simulink model "ENV_scheduled"  (R2024b)
settings: Solver=FixedStepDiscrete  StartTime=0.0  StopTime=10.0  FixedStep=0.001  RelTol=1e-3
libraries: stm32blockslib x54, canmsglib x29, simulink x7, stm32f4xxblockslib x1
(part 4 of 5)

== system ENV_scheduled/CAN Tx7 ==
  MCPInitialized : Inport  SampleTime=.001
  BBMSP0A0E : Inport  Port=2
  BBMSP0A10 : Inport  Port=3
  MTorqueVectoringFL : Inport  Port=4
  MTorqueVectoringFR : Inport  Port=5
  MTorqueVectoringRL : Inport  Port=6
  MTorqueVectoringRR : Inport  Port=7
  NTractionControlMultiplierFL : Inport  Port=8
  NTractionControlMultiplierFR : Inport  Port=9
  Bus Selector : BusSelector  OutputSignals=ID,Length,Data
  CAN Pack : canmsglib/CAN Pack  CANdbFile=C:\Users\William\Downloads\VCUSTM32\BaselineControls\CAN\CAN3_baseline.dbc  MsgList=Etas_Signals_08  MsgName=Etas_Signals_08  MsgIDType=Standard (11-bit identifier)  MsgIdentifier=2036  CANIDInput=off  MsgLength=8  Remote=off  ApplyMinMax=off  BusOutput=on  SignalInfo={'BBMSP0A0E','62','1','LE','unsigned','Standard','0','1','0','0','1';'BBMSP0A10','63','1','LE','unsigned','Standard','0','1','0','0','1';'MTorqueVectoringFL','12','12','LE','signed','Standard','0','0.1','50','-154.8','254.7';'MTorqueVectoringFR','24','12','LE','signed','Standard','0','0.1','50','-154.8','254.7';'MTorqueVectoringRL','36','12','LE','signed','Standard','0','0.1','50','-154.8','254.7';'MTorqueVectoringRR','0','12','LE','signed','Standard','0','0.1','50','-154.8','254.7';'NTractionControlMultiplierFL','55','7','LE','unsigned','Standard','0','0.01','0','0','1.27';'NTractionControlMultiplierFR','48','7','LE','unsigned','Standard','0','0.01','0','0','1.27'}
      settings: LibrarySourceBlock=stmutilitieslib/CAN Pack  DataFormat=CANdb specified signals
  MATLAB Function : MATLAB Function  TreatAsAtomicUnit=on
  Offset : Constant  Value=3  OutDataTypeStr=uint16  SampleTime=.001
  Period : Constant  Value=20  OutDataTypeStr=uint16  SampleTime=.001
  RTS : Constant  Value=0x82  OutDataTypeStr=uint8  SampleTime=.001
  SPI Controller Transfer : stm32blockslib/SPI Controller Transfer  Priority=1  SPIModuleSelect=SPI1  ClockPolarity=Low  ClockPhase=1 Edge  SPIModule=uint32(0)  Mode=Master  BusSpeed=uint32(1000000)  FirstBitToTransfer=Most significant bit (MSB)  ClockMode=0  BlockFunction=Transfer  EnableRegisterAddress=off  RegisterAddress=0  OutputDataType=uint8  OutputDataLength=1  OutputStatus=off  BlockingMode=off  Timeout=0.01  DataBits=8  UseCustomSSPin=Explicit GPIO calls  ActiveLowSSPin=Active low  Port_Select=GPIOA  Pin=4
      settings: LibrarySourceBlock=stm32h7xxblockslib/SPI Controller Transfer
  SPI Controller Transfer1 : stm32blockslib/SPI Controller Transfer  Priority=2  SPIModuleSelect=SPI1  ClockPolarity=Low  ClockPhase=1 Edge  SPIModule=uint32(0)  Mode=Master  BusSpeed=uint32(1000000)  FirstBitToTransfer=Most significant bit (MSB)  ClockMode=0  BlockFunction=Transfer  EnableRegisterAddress=off  RegisterAddress=0  OutputDataType=uint8  OutputDataLength=1  OutputStatus=off  BlockingMode=off  Timeout=0.01  DataBits=8  UseCustomSSPin=Explicit GPIO calls  ActiveLowSSPin=Active low  Port_Select=GPIOA  Pin=4
      settings: LibrarySourceBlock=stm32h7xxblockslib/SPI Controller Transfer
  TX Buffer 0 : Constant  Value=0x41  OutDataTypeStr=uint8  SampleTime=.001
  Terminator : Terminator
  Terminator1 : Terminator
  Vector Concatenate : Concatenate  NumInputs=3
  wires:
  BBMSP0A10/1 -> CAN Pack/2
  BBMSP0A0E/1 -> CAN Pack/1
  MTorqueVectoringFL/1 -> CAN Pack/3
  MTorqueVectoringFR/1 -> CAN Pack/4
  MTorqueVectoringRL/1 -> CAN Pack/5
  MTorqueVectoringRR/1 -> CAN Pack/6
  NTractionControlMultiplierFL/1 -> CAN Pack/7
  NTractionControlMultiplierFR/1 -> CAN Pack/8
  RTS/1 -> MATLAB Function/4(RTS)
  MATLAB Function/1(WriteInstruction) -> Vector Concatenate/1
  TX Buffer 0/1 -> Vector Concatenate/2
  SPI Controller Transfer1/1 -> Terminator1/1
  MATLAB Function/2(CANVector) -> Vector Concatenate/3
  Offset/1 -> MATLAB Function/6(offset)
  Bus Selector/2 -> MATLAB Function/2(Length)  "<Length>"
  Bus Selector/3 -> MATLAB Function/3(Data)  "<Data>"
  Vector Concatenate/1 -> SPI Controller Transfer/1
  MCPInitialized/1 -> MATLAB Function/7(MCPInitialized)
  Period/1 -> MATLAB Function/5(period)
  Bus Selector/1 -> MATLAB Function/1(ID)  "<ID>"
  CAN Pack/1 -> Bus Selector/1
  SPI Controller Transfer/1 -> Terminator/1
  MATLAB Function/3(RTSByte) -> SPI Controller Transfer1/1

== system ENV_scheduled/CAN Tx8 ==
  MCPInitialized : Inport  SampleTime=.001
  MDischargeLimited : Inport  Port=2
  MDriverRegenRequested : Inport  Port=3
  MRegenLimited : Inport  Port=4
  MSpinningModelFL : Inport  Port=5
  MSpinningModelFR : Inport  Port=6
  NCarState : Inport  Port=7
  rSlipRatioOptimal : Inport  Port=8
  Bus Selector : BusSelector  OutputSignals=ID,Length,Data
  CAN Pack : canmsglib/CAN Pack  CANdbFile=C:\Users\William\Downloads\VCUSTM32\BaselineControls\CAN\CAN3_baseline.dbc  MsgList=Etas_Signals_09  MsgName=Etas_Signals_09  MsgIDType=Standard (11-bit identifier)  MsgIdentifier=2037  CANIDInput=off  MsgLength=8  Remote=off  ApplyMinMax=off  BusOutput=on  SignalInfo={'MDischargeLimited','0','13','LE','unsigned','Standard','0','0.1','0','0','819.1';'MDriverRegenRequested','13','11','LE','unsigned','Standard','0','-0.1','0','-204.7','0';'MRegenLimited','30','11','LE','unsigned','Standard','0','-0.1','0','-204.7','0';'MSpinningModelFL','41','8','LE','unsigned','Standard','0','0.1','0','-Inf','Inf';'MSpinningModelFR','49','8','LE','unsigned','Standard','0','0.1','0','-Inf','Inf';'NCarState','57','7','LE','unsigned','Standard','0','1','0','0','127';'rSlipRatioOptimal','24','6','LE','unsigned','Standard','0','0.01','0','0','0.63'}
      settings: LibrarySourceBlock=stmutilitieslib/CAN Pack  DataFormat=CANdb specified signals
  MATLAB Function : MATLAB Function  TreatAsAtomicUnit=on
  Offset : Constant  Value=3  OutDataTypeStr=uint16  SampleTime=.001
  Period : Constant  Value=20  OutDataTypeStr=uint16  SampleTime=.001
  RTS : Constant  Value=0x84  OutDataTypeStr=uint8  SampleTime=.001
  SPI Controller Transfer : stm32blockslib/SPI Controller Transfer  Priority=1  SPIModuleSelect=SPI1  ClockPolarity=Low  ClockPhase=1 Edge  SPIModule=uint32(0)  Mode=Master  BusSpeed=uint32(1000000)  FirstBitToTransfer=Most significant bit (MSB)  ClockMode=0  BlockFunction=Transfer  EnableRegisterAddress=off  RegisterAddress=0  OutputDataType=uint8  OutputDataLength=1  OutputStatus=off  BlockingMode=off  Timeout=0.01  DataBits=8  UseCustomSSPin=Explicit GPIO calls  ActiveLowSSPin=Active low  Port_Select=GPIOA  Pin=4
      settings: LibrarySourceBlock=stm32h7xxblockslib/SPI Controller Transfer
  SPI Controller Transfer1 : stm32blockslib/SPI Controller Transfer  Priority=2  SPIModuleSelect=SPI1  ClockPolarity=Low  ClockPhase=1 Edge  SPIModule=uint32(0)  Mode=Master  BusSpeed=uint32(1000000)  FirstBitToTransfer=Most significant bit (MSB)  ClockMode=0  BlockFunction=Transfer  EnableRegisterAddress=off  RegisterAddress=0  OutputDataType=uint8  OutputDataLength=1  OutputStatus=off  BlockingMode=off  Timeout=0.01  DataBits=8  UseCustomSSPin=Explicit GPIO calls  ActiveLowSSPin=Active low  Port_Select=GPIOA  Pin=4
      settings: LibrarySourceBlock=stm32h7xxblockslib/SPI Controller Transfer
  TX Buffer 0 : Constant  Value=0x51  OutDataTypeStr=uint8  SampleTime=.001
  Terminator : Terminator
  Terminator1 : Terminator
  Vector Concatenate : Concatenate  NumInputs=3
  wires:
  MDriverRegenRequested/1 -> CAN Pack/2
  MDischargeLimited/1 -> CAN Pack/1
  MRegenLimited/1 -> CAN Pack/3
  MSpinningModelFL/1 -> CAN Pack/4
  MSpinningModelFR/1 -> CAN Pack/5
  NCarState/1 -> CAN Pack/6
  rSlipRatioOptimal/1 -> CAN Pack/7
  CAN Pack/1 -> Bus Selector/1
  SPI Controller Transfer/1 -> Terminator/1
  Bus Selector/1 -> MATLAB Function/1(ID)  "<ID>"
  Period/1 -> MATLAB Function/5(period)
  Bus Selector/3 -> MATLAB Function/3(Data)  "<Data>"
  Vector Concatenate/1 -> SPI Controller Transfer/1
  Bus Selector/2 -> MATLAB Function/2(Length)  "<Length>"
  Offset/1 -> MATLAB Function/6(offset)
  SPI Controller Transfer1/1 -> Terminator1/1
  MATLAB Function/2(CANVector) -> Vector Concatenate/3
  TX Buffer 0/1 -> Vector Concatenate/2
  MATLAB Function/3(RTSByte) -> SPI Controller Transfer1/1
  RTS/1 -> MATLAB Function/4(RTS)
  MCPInitialized/1 -> MATLAB Function/7(MCPInitialized)
  MATLAB Function/1(WriteInstruction) -> Vector Concatenate/1

== system ENV_scheduled/CAN Tx9 ==
  MCPInitialized : Inport  SampleTime=.001
  MSpinningModelRL : Inport  Port=2
  MSpinningModelRR : Inport  Port=3
  MTorqueDistributionFL : Inport  Port=4
  MTorqueDistributionFR : Inport  Port=5
  MTorqueDistributionRL : Inport  Port=6
  MTorqueDistributionRR : Inport  Port=7
  Bus Selector : BusSelector  OutputSignals=ID,Length,Data
  CAN Pack : canmsglib/CAN Pack  CANdbFile=C:\Users\William\Downloads\VCUSTM32\BaselineControls\CAN\CAN3_baseline.dbc  MsgList=Etas_Signals_10  MsgName=Etas_Signals_10  MsgIDType=Standard (11-bit identifier)  MsgIdentifier=2038  CANIDInput=off  MsgLength=8  Remote=off  ApplyMinMax=off  BusOutput=on  SignalInfo={'MSpinningModelRL','8','8','LE','unsigned','Standard','0','0.1','0','-Inf','Inf';'MSpinningModelRR','0','8','LE','unsigned','Standard','0','0.1','0','0','25.5';'MTorqueDistributionFL','40','12','LE','signed','Standard','0','0.1','50','-154.8','254.7';'MTorqueDistributionFR','16','12','LE','signed','Standard','0','0.1','50','-154.8','254.7';'MTorqueDistributionRL','52','12','LE','signed','Standard','0','0.1','50','-154.8','254.7';'MTorqueDistributionRR','28','12','LE','signed','Standard','0','0.1','50','-154.8','254.7'}
      settings: LibrarySourceBlock=stmutilitieslib/CAN Pack  DataFormat=CANdb specified signals
  MATLAB Function : MATLAB Function  TreatAsAtomicUnit=on
  Offset : Constant  Value=4  OutDataTypeStr=uint16  SampleTime=.001
  Period : Constant  Value=20  OutDataTypeStr=uint16  SampleTime=.001
  RTS : Constant  Value=0x81  OutDataTypeStr=uint8  SampleTime=.001
  SPI Controller Transfer : stm32blockslib/SPI Controller Transfer  Priority=1  SPIModuleSelect=SPI1  ClockPolarity=Low  ClockPhase=1 Edge  SPIModule=uint32(0)  Mode=Master  BusSpeed=uint32(1000000)  FirstBitToTransfer=Most significant bit (MSB)  ClockMode=0  BlockFunction=Transfer  EnableRegisterAddress=off  RegisterAddress=0  OutputDataType=uint8  OutputDataLength=1  OutputStatus=off  BlockingMode=off  Timeout=0.01  DataBits=8  UseCustomSSPin=Explicit GPIO calls  ActiveLowSSPin=Active low  Port_Select=GPIOA  Pin=4
      settings: LibrarySourceBlock=stm32h7xxblockslib/SPI Controller Transfer
  SPI Controller Transfer1 : stm32blockslib/SPI Controller Transfer  Priority=2  SPIModuleSelect=SPI1  ClockPolarity=Low  ClockPhase=1 Edge  SPIModule=uint32(0)  Mode=Master  BusSpeed=uint32(1000000)  FirstBitToTransfer=Most significant bit (MSB)  ClockMode=0  BlockFunction=Transfer  EnableRegisterAddress=off  RegisterAddress=0  OutputDataType=uint8  OutputDataLength=1  OutputStatus=off  BlockingMode=off  Timeout=0.01  DataBits=8  UseCustomSSPin=Explicit GPIO calls  ActiveLowSSPin=Active low  Port_Select=GPIOA  Pin=4
      settings: LibrarySourceBlock=stm32h7xxblockslib/SPI Controller Transfer
  TX Buffer 0 : Constant  Value=0x31  OutDataTypeStr=uint8  SampleTime=.001
  Terminator : Terminator
  Terminator1 : Terminator
  Vector Concatenate : Concatenate  NumInputs=3
  wires:
  MSpinningModelRR/1 -> CAN Pack/2
  MSpinningModelRL/1 -> CAN Pack/1
  MTorqueDistributionFL/1 -> CAN Pack/3
  MTorqueDistributionFR/1 -> CAN Pack/4
  MTorqueDistributionRL/1 -> CAN Pack/5
  MTorqueDistributionRR/1 -> CAN Pack/6
  CAN Pack/1 -> Bus Selector/1
  Vector Concatenate/1 -> SPI Controller Transfer/1
  Bus Selector/1 -> MATLAB Function/1(ID)  "<ID>"
  Bus Selector/2 -> MATLAB Function/2(Length)  "<Length>"
  TX Buffer 0/1 -> Vector Concatenate/2
  MATLAB Function/2(CANVector) -> Vector Concatenate/3
  MATLAB Function/3(RTSByte) -> SPI Controller Transfer1/1
  SPI Controller Transfer1/1 -> Terminator1/1
  RTS/1 -> MATLAB Function/4(RTS)
  Period/1 -> MATLAB Function/5(period)
  MCPInitialized/1 -> MATLAB Function/7(MCPInitialized)
  MATLAB Function/1(WriteInstruction) -> Vector Concatenate/1
  Bus Selector/3 -> MATLAB Function/3(Data)  "<Data>"
  Offset/1 -> MATLAB Function/6(offset)
  SPI Controller Transfer/1 -> Terminator/1

== system ENV_scheduled/Subsystem ==
  Detect Increase : simulink/Logic and Bit Operations/Detect Increase  vinit=0.0  OutDataTypeStr=boolean
  Initialize : Subsystem  TreatAsAtomicUnit=on
  MCPInit : Subsystem  TreatAsAtomicUnit=on
  Step1 : Step  SampleTime=0.001
  Step2 : Step  SampleTime=0.001
  Unit Delay : UnitDelay  SampleTime=0.001  HasFrameUpgradeWarning=on
  MCPInitialized : Outport  SampleTime=0.001
  wires:
  Step1/1 -> Detect Increase/1
  Unit Delay/1 -> Initialize/Enable
  Detect Increase/1 -> MCPInit/Enable
  Step2/1 -> Unit Delay/1
  Initialize/1(MCPInitialized) -> MCPInitialized/1

== system ENV_scheduled/gLat ==
  In1 : Inport
  Compare To Constant : simulink/Logic and Bit Operations/Compare To Constant  relop=>=  const=-0.1  OutDataTypeStr=boolean
  Compare To Constant1 : simulink/Logic and Bit Operations/Compare To Constant  relop=<=  const=0.1  OutDataTypeStr=boolean
  Memory : Memory  InheritSampleTime=on
  OR : Logic  AllPortsSameDT=off  OutDataTypeStr=boolean
  Switch : Switch  Criteria=u2 ~= 0  SaturateOnIntegerOverflow=off  InputSameDT=off
  Out1 : Outport  VectorParamsAs1DForOutWhenUnconnected=off
  wires:
  Switch/1 -> Memory/1, Out1/1
  In1/1 -> Switch/3, Compare To Constant1/1, Compare To Constant/1
  Memory/1 -> Switch/1
  Compare To Constant/1 -> OR/1
  Compare To Constant1/1 -> OR/2
  OR/1 -> Switch/2

== system ENV_scheduled/gLong ==
  In1 : Inport
  Compare To Constant : simulink/Logic and Bit Operations/Compare To Constant  relop=>=  const=9.9  OutDataTypeStr=boolean
  Compare To Constant1 : simulink/Logic and Bit Operations/Compare To Constant  relop=<=  const=10.1  OutDataTypeStr=boolean
  Memory : Memory  InheritSampleTime=on
  OR : Logic  AllPortsSameDT=off  OutDataTypeStr=boolean
  Switch : Switch  Criteria=u2 ~= 0  SaturateOnIntegerOverflow=off  InputSameDT=off
  Out1 : Outport  VectorParamsAs1DForOutWhenUnconnected=off
  wires:
  Memory/1 -> Switch/1
  Switch/1 -> Out1/1, Memory/1
  In1/1 -> Compare To Constant1/1, Switch/3, Compare To Constant/1
  Compare To Constant/1 -> OR/1
  Compare To Constant1/1 -> OR/2
  OR/1 -> Switch/2

== system ENV_scheduled/Subsystem/Initialize ==
  Enable : EnablePort
  Constant : Constant  OutDataTypeStr=boolean
  MCPInitialized : Outport  SampleTime=0.001
  wires:
  Constant/1 -> MCPInitialized/1

== system ENV_scheduled/Subsystem/MCPInit ==
  note: 0x02, 0x2A, 0x40 | 0x02, 0x29, 0x9B | 0x02, 0x28, 0x83 | 0x02, 0x0F, 0x14
  Enable : EnablePort
  " 000: normal mode, 0: don't abort pending transmit buffers, 0: one-shot disabled, 0: CLKOUT disabled, 00: sysclk/1 | 0000 0000 | 0x00" : Constant  Value=[0x02, 0x0F, 0x00]  OutDataTypeStr=uint8
  CNF1 : Constant  Value=[0x02, 0x2A, 0xC0]  OutDataTypeStr=uint8
  CNF2 : Constant  Value=[0x02, 0x29, 0x99]  OutDataTypeStr=uint8
  CNF3 : Constant  Value=[0x02, 0x28, 0x02]  OutDataTypeStr=uint8
  Enter Configuration Mode : Constant  Value=0xc0  OutDataTypeStr=uint8
  SPI Controller Transfer : stm32blockslib/SPI Controller Transfer  Priority=4  SPIModuleSelect=SPI1  ClockPolarity=Low  ClockPhase=1 Edge  SPIModule=uint32(0)  Mode=Master  BusSpeed=uint32(1000000)  FirstBitToTransfer=Most significant bit (MSB)  ClockMode=0  BlockFunction=Transfer  EnableRegisterAddress=off  RegisterAddress=0  OutputDataType=uint8  OutputDataLength=1  OutputStatus=off  BlockingMode=on  Timeout=0.01  DataBits=8  UseCustomSSPin=Explicit GPIO calls  ActiveLowSSPin=Active low  Port_Select=GPIOA  Pin=4
      settings: LibrarySourceBlock=stm32h7xxblockslib/SPI Controller Transfer
  SPI Controller Transfer1 : stm32blockslib/SPI Controller Transfer  Priority=5  SPIModuleSelect=SPI1  ClockPolarity=Low  ClockPhase=1 Edge  SPIModule=uint32(0)  Mode=Master  BusSpeed=uint32(1000000)  FirstBitToTransfer=Most significant bit (MSB)  ClockMode=0  BlockFunction=Transfer  EnableRegisterAddress=off  RegisterAddress=0  OutputDataType=uint8  OutputDataLength=1  OutputStatus=off  BlockingMode=on  Timeout=0.01  DataBits=8  UseCustomSSPin=Explicit GPIO calls  ActiveLowSSPin=Active low  Port_Select=GPIOA  Pin=4
      settings: LibrarySourceBlock=stm32h7xxblockslib/SPI Controller Transfer
  SPI Controller Transfer2 : stm32blockslib/SPI Controller Transfer  Priority=6  SPIModuleSelect=SPI1  ClockPolarity=Low  ClockPhase=1 Edge  SPIModule=uint32(0)  Mode=Master  BusSpeed=uint32(1000000)  FirstBitToTransfer=Most significant bit (MSB)  ClockMode=0  BlockFunction=Transfer  EnableRegisterAddress=off  RegisterAddress=0  OutputDataType=uint8  OutputDataLength=1  OutputStatus=off  BlockingMode=on  Timeout=0.01  DataBits=8  UseCustomSSPin=Explicit GPIO calls  ActiveLowSSPin=Active low  Port_Select=GPIOA  Pin=4
      settings: LibrarySourceBlock=stm32h7xxblockslib/SPI Controller Transfer
  SPI Controller Transfer3 : stm32blockslib/SPI Controller Transfer  Priority=7  SPIModuleSelect=SPI1  ClockPolarity=Low  ClockPhase=1 Edge  SPIModule=uint32(0)  Mode=Master  BusSpeed=uint32(1000000)  FirstBitToTransfer=Most significant bit (MSB)  ClockMode=0  BlockFunction=Transfer  EnableRegisterAddress=off  RegisterAddress=0  OutputDataType=uint8  OutputDataLength=1  OutputStatus=off  BlockingMode=on  Timeout=0.01  DataBits=8  UseCustomSSPin=Explicit GPIO calls  ActiveLowSSPin=Active low  Port_Select=GPIOA  Pin=4
      settings: LibrarySourceBlock=stm32h7xxblockslib/SPI Controller Transfer
  SPI Controller Transfer4 : stm32blockslib/SPI Controller Transfer  Priority=8  SPIModuleSelect=SPI1  ClockPolarity=Low  ClockPhase=1 Edge  SPIModule=uint32(0)  Mode=Master  BusSpeed=uint32(1000000)  FirstBitToTransfer=Most significant bit (MSB)  ClockMode=0  BlockFunction=Transfer  EnableRegisterAddress=off  RegisterAddress=0  OutputDataType=uint8  OutputDataLength=1  OutputStatus=off  BlockingMode=on  Timeout=0.01  DataBits=8  UseCustomSSPin=Explicit GPIO calls  ActiveLowSSPin=Active low  Port_Select=GPIOA  Pin=4
      settings: LibrarySourceBlock=stm32h7xxblockslib/SPI Controller Transfer
  Terminator{,1..4} (5 alike) : Terminator
  wires:
  SPI Controller Transfer/1 -> Terminator/1
  Enter Configuration Mode/1 -> SPI Controller Transfer/1
  CNF1/1 -> SPI Controller Transfer1/1
  SPI Controller Transfer1/1 -> Terminator1/1
  CNF2/1 -> SPI Controller Transfer2/1
  SPI Controller Transfer2/1 -> Terminator2/1
  CNF3/1 -> SPI Controller Transfer3/1
  SPI Controller Transfer3/1 -> Terminator3/1
  " 000: normal mode, 0: don't abort pending transmit buffers, 0: one-shot disabled, 0: CLKOUT disabled, 00: sysclk/1 | 0000 0000 | 0x00"/1 -> SPI Controller Transfer4/1
  SPI Controller Transfer4/1 -> Terminator4/1

== matlab function ENV_scheduled/CAN Tx2/MATLAB Function ==
  settings: updateMethod=DISCRETE  sampleTime=.001
  data: WriteInstruction output; ID input uint32; CANVector output uint8; Length input uint8; Data input uint8; RTS input; RTSByte output; period input; offset input; MCPInitialized input
function [WriteInstruction, CANVector, RTSByte] = ConvertToVector(ID, Length, Data, RTS, period, offset, MCPInitialized)
%#codegen
persistent count;
if isempty(count)
    count = uint16(0);
end

if MCPInitialized
    if count == uint16(7)
        id_u16 = uint16(ID);
        CANVector = zeros(1,13,'uint8');
        CANVector(1) = uint8(bitshift(id_u16, -3));
        CANVector(2) = uint8(bitshift(bitand(id_u16, uint16(7)), 5));
        CANVector(3) = uint8(0);
        CANVector(4) = uint8(0);
        CANVector(5) = bitand(uint8(Length), uint8(15));
        for i = 1:8
            CANVector(5+i) = uint8(Data(i));
        end
        RTSByte = uint8(RTS);
        WriteInstruction = uint8(0x02);
    else
        CANVector = zeros(1,13,'uint8');
        RTSByte = uint8(RTS);
        WriteInstruction = uint8(0x03);
    end

    count = count + uint16(1);
    if count >= uint16(period)
        count = uint16(0);
    end
else
    CANVector = zeros(1,13,'uint8');
    RTSByte = uint8(0x03);
    WriteInstruction = uint8(0x03);
    % don't increment count while MCP not ready
end

== matlab function ENV_scheduled/CAN Tx3/MATLAB Function ==
  settings: updateMethod=DISCRETE  sampleTime=.001
  data: WriteInstruction output; ID input uint32; CANVector output uint8; Length input uint8; Data input uint8; RTS input; RTSByte output; period input; offset input; MCPInitialized input
function [WriteInstruction, CANVector, RTSByte] = ConvertToVector(ID, Length, Data, RTS, period, offset, MCPInitialized)
%#codegen
persistent count;
if isempty(count)
    count = uint16(0);
end

if MCPInitialized
    if count == uint16(offset)
        id_u16 = uint16(ID);
        CANVector = zeros(1,13,'uint8');
        CANVector(1) = uint8(bitshift(id_u16, -3));
        CANVector(2) = uint8(bitshift(bitand(id_u16, uint16(7)), 5));
        CANVector(3) = uint8(0);
        CANVector(4) = uint8(0);
        CANVector(5) = bitand(uint8(Length), uint8(15));
        for i = 1:8
            CANVector(5+i) = uint8(Data(i));
        end
        RTSByte = uint8(RTS);
        WriteInstruction = uint8(0x02);
    else
        CANVector = zeros(1,13,'uint8');
        RTSByte = uint8(RTS);
        WriteInstruction = uint8(0x03);
    end

    count = count + uint16(1);
    if count >= uint16(period)
        count = uint16(0);
    end
else
    CANVector = zeros(1,13,'uint8');
    RTSByte = uint8(0x03);
    WriteInstruction = uint8(0x03);
    % don't increment count while MCP not ready
end

== matlab function ENV_scheduled/CAN Tx4/MATLAB Function ==
  settings: updateMethod=DISCRETE  sampleTime=.001
  data: WriteInstruction output; ID input uint32; CANVector output uint8; Length input uint8; Data input uint8; RTS input; RTSByte output; period input; offset input; MCPInitialized input
function [WriteInstruction, CANVector, RTSByte] = ConvertToVector(ID, Length, Data, RTS, period, offset, MCPInitialized)
%#codegen
persistent count;
if isempty(count)
    count = uint16(0);
end

if MCPInitialized
    if count == uint16(7)
        id_u16 = uint16(ID);
        CANVector = zeros(1,13,'uint8');
        CANVector(1) = uint8(bitshift(id_u16, -3));
        CANVector(2) = uint8(bitshift(bitand(id_u16, uint16(7)), 5));
        CANVector(3) = uint8(0);
        CANVector(4) = uint8(0);
        CANVector(5) = bitand(uint8(Length), uint8(15));
        for i = 1:8
            CANVector(5+i) = uint8(Data(i));
        end
        RTSByte = uint8(RTS);
        WriteInstruction = uint8(0x02);
    else
        CANVector = zeros(1,13,'uint8');
        RTSByte = uint8(RTS);
        WriteInstruction = uint8(0x03);
    end

    count = count + uint16(1);
    if count >= uint16(period)
        count = uint16(0);
    end
else
    CANVector = zeros(1,13,'uint8');
    RTSByte = uint8(0x03);
    WriteInstruction = uint8(0x03);
    % don't increment count while MCP not ready
end

== matlab function ENV_scheduled/CAN Tx5/MATLAB Function ==
  settings: updateMethod=DISCRETE  sampleTime=.001
  data: WriteInstruction output; ID input uint32; CANVector output uint8; Length input uint8; Data input uint8; RTS input; RTSByte output; period input; offset input; MCPInitialized input
function [WriteInstruction, CANVector, RTSByte] = ConvertToVector(ID, Length, Data, RTS, period, offset, MCPInitialized)
%#codegen
persistent count;
if isempty(count)
    count = uint16(0);
end

if MCPInitialized
    if count == uint16(1)
        id_u16 = uint16(ID);
        CANVector = zeros(1,13,'uint8');
        CANVector(1) = uint8(bitshift(id_u16, -3));
        CANVector(2) = uint8(bitshift(bitand(id_u16, uint16(7)), 5));
        CANVector(3) = uint8(0);
        CANVector(4) = uint8(0);
        CANVector(5) = bitand(uint8(Length), uint8(15));
        for i = 1:8
            CANVector(5+i) = uint8(Data(i));
        end
        RTSByte = uint8(RTS);
        WriteInstruction = uint8(0x02);
    else
        CANVector = zeros(1,13,'uint8');
        RTSByte = uint8(RTS);
        WriteInstruction = uint8(0x03);
    end

    count = count + uint16(1);
    if count >= uint16(period)
        count = uint16(0);
    end
else
    CANVector = zeros(1,13,'uint8');
    RTSByte = uint8(0x03);
    WriteInstruction = uint8(0x03);
    % don't increment count while MCP not ready
end

== matlab function ENV_scheduled/CAN Tx6/MATLAB Function ==
  settings: updateMethod=DISCRETE  sampleTime=.001
  data: WriteInstruction output; ID input uint32; CANVector output uint8; Length input uint8; Data input uint8; RTS input; RTSByte output; period input; offset input; MCPInitialized input
function [WriteInstruction, CANVector, RTSByte] = ConvertToVector(ID, Length, Data, RTS, period, offset, MCPInitialized)
%#codegen
persistent count;
if isempty(count)
    count = uint16(0);
end

if MCPInitialized
    if count == uint16(offset)
        id_u16 = uint16(ID);
        CANVector = zeros(1,13,'uint8');
        CANVector(1) = uint8(bitshift(id_u16, -3));
        CANVector(2) = uint8(bitshift(bitand(id_u16, uint16(7)), 5));
        CANVector(3) = uint8(0);
        CANVector(4) = uint8(0);
        CANVector(5) = bitand(uint8(Length), uint8(15));
        for i = 1:8
            CANVector(5+i) = uint8(Data(i));
        end
        RTSByte = uint8(RTS);
        WriteInstruction = uint8(0x02);
    else
        CANVector = zeros(1,13,'uint8');
        RTSByte = uint8(RTS);
        WriteInstruction = uint8(0x03);
    end

    count = count + uint16(1);
    if count >= uint16(period)
        count = uint16(0);
    end
else
    CANVector = zeros(1,13,'uint8');
    RTSByte = uint8(0x03);
    WriteInstruction = uint8(0x03);
    % don't increment count while MCP not ready
end

== matlab function ENV_scheduled/CAN Tx7/MATLAB Function ==
  settings: updateMethod=DISCRETE  sampleTime=.001
  data: WriteInstruction output; ID input uint32; CANVector output uint8; Length input uint8; Data input uint8; RTS input; RTSByte output; period input; offset input; MCPInitialized input
function [WriteInstruction, CANVector, RTSByte] = ConvertToVector(ID, Length, Data, RTS, period, offset, MCPInitialized)
%#codegen
persistent count;
if isempty(count)
    count = uint16(0);
end

if MCPInitialized
    if count == uint16(offset)
        id_u16 = uint16(ID);
        CANVector = zeros(1,13,'uint8');
        CANVector(1) = uint8(bitshift(id_u16, -3));
        CANVector(2) = uint8(bitshift(bitand(id_u16, uint16(7)), 5));
        CANVector(3) = uint8(0);
        CANVector(4) = uint8(0);
        CANVector(5) = bitand(uint8(Length), uint8(15));
        for i = 1:8
            CANVector(5+i) = uint8(Data(i));
        end
        RTSByte = uint8(RTS);
        WriteInstruction = uint8(0x02);
    else
        CANVector = zeros(1,13,'uint8');
        RTSByte = uint8(RTS);
        WriteInstruction = uint8(0x03);
    end

    count = count + uint16(1);
    if count >= uint16(period)
        count = uint16(0);
    end
else
    CANVector = zeros(1,13,'uint8');
    RTSByte = uint8(0x03);
    WriteInstruction = uint8(0x03);
    % don't increment count while MCP not ready
end

== matlab function ENV_scheduled/CAN Tx8/MATLAB Function ==
  settings: updateMethod=DISCRETE  sampleTime=.001
  data: WriteInstruction output; ID input uint32; CANVector output uint8; Length input uint8; Data input uint8; RTS input; RTSByte output; period input; offset input; MCPInitialized input
function [WriteInstruction, CANVector, RTSByte] = ConvertToVector(ID, Length, Data, RTS, period, offset, MCPInitialized)
%#codegen
persistent count;
if isempty(count)
    count = uint16(0);
end

if MCPInitialized
    if count == uint16(offset)
        id_u16 = uint16(ID);
        CANVector = zeros(1,13,'uint8');
        CANVector(1) = uint8(bitshift(id_u16, -3));
        CANVector(2) = uint8(bitshift(bitand(id_u16, uint16(7)), 5));
        CANVector(3) = uint8(0);
        CANVector(4) = uint8(0);
        CANVector(5) = bitand(uint8(Length), uint8(15));
        for i = 1:8
            CANVector(5+i) = uint8(Data(i));
        end
        RTSByte = uint8(RTS);
        WriteInstruction = uint8(0x02);
    else
        CANVector = zeros(1,13,'uint8');
        RTSByte = uint8(RTS);
        WriteInstruction = uint8(0x03);
    end

    count = count + uint16(1);
    if count >= uint16(period)
        count = uint16(0);
    end
else
    CANVector = zeros(1,13,'uint8');
    RTSByte = uint8(0x03);
    WriteInstruction = uint8(0x03);
    % don't increment count while MCP not ready
end

== matlab function ENV_scheduled/CAN Tx1/MATLAB Function ==
  settings: updateMethod=DISCRETE  sampleTime=.001
  data: WriteInstruction output; ID input uint32; CANVector output uint8; Length input uint8; Data input uint8; RTS input; RTSByte output; period input; offset input; MCPInitialized input
function [WriteInstruction, CANVector, RTSByte] = ConvertToVector(ID, Length, Data, RTS, period, offset, MCPInitialized)
%#codegen
persistent count;
if isempty(count)
    count = uint16(0);
end

if MCPInitialized
    if count == uint16(offset)
        id_u16 = uint16(ID);
        CANVector = zeros(1,13,'uint8');
        CANVector(1) = uint8(bitshift(id_u16, -3));
        CANVector(2) = uint8(bitshift(bitand(id_u16, uint16(7)), 5));
        CANVector(3) = uint8(0);
        CANVector(4) = uint8(0);
        CANVector(5) = bitand(uint8(Length), uint8(15));
        for i = 1:8
            CANVector(5+i) = uint8(Data(i));
        end
        RTSByte = uint8(RTS);
        WriteInstruction = uint8(0x02);
    else
        CANVector = zeros(1,13,'uint8');
        RTSByte = uint8(0x03);
        WriteInstruction = uint8(0x03);
    end

    count = count + uint16(1);
    if count >= uint16(period)
        count = uint16(0);
    end
else
    CANVector = zeros(1,13,'uint8');
    RTSByte = uint8(0x03);
    WriteInstruction = uint8(0x03);
    % don't increment count while MCP not ready
end

== matlab function ENV_scheduled/CAN Tx9/MATLAB Function ==
  settings: updateMethod=DISCRETE  sampleTime=.001
  data: WriteInstruction output; ID input uint32; CANVector output uint8; Length input uint8; Data input uint8; RTS input; RTSByte output; period input; offset input; MCPInitialized input
function [WriteInstruction, CANVector, RTSByte] = ConvertToVector(ID, Length, Data, RTS, period, offset, MCPInitialized)
%#codegen
persistent count;
if isempty(count)
    count = uint16(0);
end

if MCPInitialized
    if count == uint16(offset)
        id_u16 = uint16(ID);
        CANVector = zeros(1,13,'uint8');
        CANVector(1) = uint8(bitshift(id_u16, -3));
        CANVector(2) = uint8(bitshift(bitand(id_u16, uint16(7)), 5));
        CANVector(3) = uint8(0);
        CANVector(4) = uint8(0);
        CANVector(5) = bitand(uint8(Length), uint8(15));
        for i = 1:8
            CANVector(5+i) = uint8(Data(i));
        end
        RTSByte = uint8(RTS);
        WriteInstruction = uint8(0x02);
    else
        CANVector = zeros(1,13,'uint8');
        RTSByte = uint8(RTS);
        WriteInstruction = uint8(0x03);
    end

    count = count + uint16(1);
    if count >= uint16(period)
        count = uint16(0);
    end
else
    CANVector = zeros(1,13,'uint8');
    RTSByte = uint8(0x03);
    WriteInstruction = uint8(0x03);
    % don't increment count while MCP not ready
end

== matlab function ENV_scheduled/CAN Tx10/MATLAB Function ==
  settings: updateMethod=DISCRETE  sampleTime=.001
  data: WriteInstruction output; ID input uint32; CANVector output uint8; Length input uint8; Data input uint8; RTS input; RTSByte output; period input; offset input; MCPInitialized input
function [WriteInstruction, CANVector, RTSByte] = ConvertToVector(ID, Length, Data, RTS, period, offset, MCPInitialized)
%#codegen
persistent count;
if isempty(count)
    count = uint16(0);
end

if MCPInitialized
    if count == uint16(offset)
        id_u16 = uint16(ID);
        CANVector = zeros(1,13,'uint8');
        CANVector(1) = uint8(bitshift(id_u16, -3));
        CANVector(2) = uint8(bitshift(bitand(id_u16, uint16(7)), 5));
        CANVector(3) = uint8(0);
        CANVector(4) = uint8(0);
        CANVector(5) = bitand(uint8(Length), uint8(15));
        for i = 1:8
            CANVector(5+i) = uint8(Data(i));
        end
        RTSByte = uint8(RTS);
        WriteInstruction = uint8(0x02);
    else
        CANVector = zeros(1,13,'uint8');
        RTSByte = uint8(RTS);
        WriteInstruction = uint8(0x03);
    end

    count = count + uint16(1);
    if count >= uint16(period)
        count = uint16(0);
    end
else
    CANVector = zeros(1,13,'uint8');
    RTSByte = uint8(0x03);
    WriteInstruction = uint8(0x03);
    % don't increment count while MCP not ready
end

== matlab function ENV_scheduled/CAN Tx11/MATLAB Function ==
  settings: updateMethod=DISCRETE  sampleTime=.001
  data: WriteInstruction output; ID input uint32; CANVector output uint8; Length input uint8; Data input uint8; RTS input; RTSByte output; period input; offset input; MCPInitialized input
function [WriteInstruction, CANVector, RTSByte] = ConvertToVector(ID, Length, Data, RTS, period, offset, MCPInitialized)
%#codegen
persistent count;
if isempty(count)
    count = uint16(0);
end

if MCPInitialized
    if count == uint16(offset)
        id_u16 = uint16(ID);
        CANVector = zeros(1,13,'uint8');
        CANVector(1) = uint8(bitshift(id_u16, -3));
        CANVector(2) = uint8(bitshift(bitand(id_u16, uint16(7)), 5));
        CANVector(3) = uint8(0);
        CANVector(4) = uint8(0);
        CANVector(5) = bitand(uint8(Length), uint8(15));
        for i = 1:8
            CANVector(5+i) = uint8(Data(i));
        end
        RTSByte = uint8(RTS);
        WriteInstruction = uint8(0x02);
    else
        CANVector = zeros(1,13,'uint8');
        RTSByte = uint8(RTS);
        WriteInstruction = uint8(0x03);
    end

    count = count + uint16(1);
    if count >= uint16(period)
        count = uint16(0);
    end
else
    CANVector = zeros(1,13,'uint8');
    RTSByte = uint8(0x03);
    WriteInstruction = uint8(0x03);
    % don't increment count while MCP not ready
end

== matlab function ENV_scheduled/CAN Tx12/MATLAB Function ==
  settings: updateMethod=DISCRETE  sampleTime=.001
  data: WriteInstruction output; ID input uint32; CANVector output uint8; Length input uint8; Data input uint8; RTS input; RTSByte output; period input; offset input; MCPInitialized input
function [WriteInstruction, CANVector, RTSByte] = ConvertToVector(ID, Length, Data, RTS, period, offset, MCPInitialized)
%#codegen
persistent count;
if isempty(count)
    count = uint16(0);
end

if MCPInitialized
    if count == uint16(2)
        id_u16 = uint16(ID);
        CANVector = zeros(1,13,'uint8');
        CANVector(1) = uint8(bitshift(id_u16, -3));
        CANVector(2) = uint8(bitshift(bitand(id_u16, uint16(7)), 5));
        CANVector(3) = uint8(0);
        CANVector(4) = uint8(0);
        CANVector(5) = bitand(uint8(Length), uint8(15));
        for i = 1:8
            CANVector(5+i) = uint8(Data(i));
        end
        RTSByte = uint8(RTS);
        WriteInstruction = uint8(0x02);
    else
        CANVector = zeros(1,13,'uint8');
        RTSByte = uint8(RTS);
        WriteInstruction = uint8(0x03);
    end

    count = count + uint16(1);
    if count >= uint16(period)
        count = uint16(0);
    end
else
    CANVector = zeros(1,13,'uint8');
    RTSByte = uint8(0x03);
    WriteInstruction = uint8(0x03);
    % don't increment count while MCP not ready
end

== matlab function ENV_scheduled/CAN Tx13/MATLAB Function ==
  settings: updateMethod=DISCRETE  sampleTime=.001
  data: WriteInstruction output; ID input uint32; CANVector output uint8; Length input uint8; Data input uint8; RTS input; RTSByte output; period input; offset input; MCPInitialized input
function [WriteInstruction, CANVector, RTSByte] = ConvertToVector(ID, Length, Data, RTS, period, offset, MCPInitialized)
%#codegen
persistent count;
if isempty(count)
    count = uint16(0);
end

if MCPInitialized
    if count == uint16(1)
        id_u16 = uint16(ID);
        CANVector = zeros(1,13,'uint8');
        CANVector(1) = uint8(bitshift(id_u16, -3));
        CANVector(2) = uint8(bitshift(bitand(id_u16, uint16(7)), 5));
        CANVector(3) = uint8(0);
        CANVector(4) = uint8(0);
        CANVector(5) = bitand(uint8(Length), uint8(15));
        for i = 1:8
            CANVector(5+i) = uint8(Data(i));
        end
        RTSByte = uint8(RTS);
        WriteInstruction = uint8(0x02);
    else
        CANVector = zeros(1,13,'uint8');
        RTSByte = uint8(RTS);
        WriteInstruction = uint8(0x03);
    end

    count = count + uint16(1);
    if count >= uint16(period)
        count = uint16(0);
    end
else
    CANVector = zeros(1,13,'uint8');
    RTSByte = uint8(0x03);
    WriteInstruction = uint8(0x03);
    % don't increment count while MCP not ready
end

== matlab function ENV_scheduled/CAN Tx14/MATLAB Function ==
  settings: updateMethod=DISCRETE  sampleTime=.001
  data: WriteInstruction output; ID input uint32; CANVector output uint8; Length input uint8; Data input uint8; RTS input; RTSByte output; period input; offset input; MCPInitialized input
function [WriteInstruction, CANVector, RTSByte] = ConvertToVector(ID, Length, Data, RTS, period, offset, MCPInitialized)
%#codegen
persistent count;
if isempty(count)
    count = uint16(0);
end

if MCPInitialized
    if count == uint16(offset)
        id_u16 = uint16(ID);
        CANVector = zeros(1,13,'uint8');
        CANVector(1) = uint8(bitshift(id_u16, -3));
        CANVector(2) = uint8(bitshift(bitand(id_u16, uint16(7)), 5));
        CANVector(3) = uint8(0);
        CANVector(4) = uint8(0);
        CANVector(5) = bitand(uint8(Length), uint8(15));
        for i = 1:8
            CANVector(5+i) = uint8(Data(i));
        end
        RTSByte = uint8(RTS);
        WriteInstruction = uint8(0x02);
    else
        CANVector = zeros(1,13,'uint8');
        RTSByte = uint8(RTS);
        WriteInstruction = uint8(0x03);
    end

    count = count + uint16(1);
    if count >= uint16(period)
        count = uint16(0);
    end
else
    CANVector = zeros(1,13,'uint8');
    RTSByte = uint8(0x03);
    WriteInstruction = uint8(0x03);
    % don't increment count while MCP not ready
end

== matlab function ENV_scheduled/CAN Tx17/MATLAB Function ==
  settings: updateMethod=DISCRETE  sampleTime=.001
  data: WriteInstruction output; ID input uint32; CANVector output uint8; Length input uint8; Data input uint8; RTS input; RTSByte output; period input; offset input; MCPInitialized input
function [WriteInstruction, CANVector, RTSByte] = ConvertToVector(ID, Length, Data, RTS, period, offset, MCPInitialized)
%#codegen
persistent count;
if isempty(count)
    count = uint16(0);
end

if MCPInitialized
    if count == uint16(offset)
        id_u16 = uint16(ID);
        CANVector = zeros(1,13,'uint8');
        CANVector(1) = uint8(bitshift(id_u16, -3));
        CANVector(2) = uint8(bitshift(bitand(id_u16, uint16(7)), 5));
        CANVector(3) = uint8(0);
        CANVector(4) = uint8(0);
        CANVector(5) = bitand(uint8(Length), uint8(15));
        for i = 1:8
            CANVector(5+i) = uint8(Data(i));
        end
        RTSByte = uint8(RTS);
        WriteInstruction = uint8(0x02);
    else
        CANVector = zeros(1,13,'uint8');
        RTSByte = uint8(RTS);
        WriteInstruction = uint8(0x03);
    end

    count = count + uint16(1);
    if count >= uint16(period)
        count = uint16(0);
    end
else
    CANVector = zeros(1,13,'uint8');
    RTSByte = uint8(0x03);
    WriteInstruction = uint8(0x03);
    % don't increment count while MCP not ready
end

== matlab function ENV_scheduled/CAN Tx16/MATLAB Function ==
  settings: updateMethod=DISCRETE  sampleTime=.001
  data: WriteInstruction output; ID input uint32; CANVector output uint8; Length input uint8; Data input uint8; RTS input; RTSByte output; period input; offset input; MCPInitialized input
function [WriteInstruction, CANVector, RTSByte] = ConvertToVector(ID, Length, Data, RTS, period, offset, MCPInitialized)
%#codegen
persistent count;
if isempty(count)
    count = uint16(0);
end

if MCPInitialized
    if count == uint16(offset)
        id_u16 = uint16(ID);
        CANVector = zeros(1,13,'uint8');
        CANVector(1) = uint8(bitshift(id_u16, -3));
        CANVector(2) = uint8(bitshift(bitand(id_u16, uint16(7)), 5));
        CANVector(3) = uint8(0);
        CANVector(4) = uint8(0);
        CANVector(5) = bitand(uint8(Length), uint8(15));
        for i = 1:8
            CANVector(5+i) = uint8(Data(i));
        end
        RTSByte = uint8(RTS);
        WriteInstruction = uint8(0x02);
    else
        CANVector = zeros(1,13,'uint8');
        RTSByte = uint8(RTS);
        WriteInstruction = uint8(0x03);
    end

    count = count + uint16(1);
    if count >= uint16(period)
        count = uint16(0);
    end
else
    CANVector = zeros(1,13,'uint8');
    RTSByte = uint8(0x03);
    WriteInstruction = uint8(0x03);
    % don't increment count while MCP not ready
end

== matlab function ENV_scheduled/CAN Tx18/MATLAB Function ==
  settings: updateMethod=DISCRETE  sampleTime=.001
  data: WriteInstruction output; ID input uint32; CANVector output uint8; Length input uint8; Data input uint8; RTS input; RTSByte output; period input; offset input; MCPInitialized input
function [WriteInstruction, CANVector, RTSByte] = ConvertToVector(ID, Length, Data, RTS, period, offset, MCPInitialized)
%#codegen
persistent count;
if isempty(count)
    count = uint16(0);
end

if MCPInitialized
    if count == uint16(offset)
        id_u16 = uint16(ID);
        CANVector = zeros(1,13,'uint8');
        CANVector(1) = uint8(bitshift(id_u16, -3));
        CANVector(2) = uint8(bitshift(bitand(id_u16, uint16(7)), 5));
        CANVector(3) = uint8(0);
        CANVector(4) = uint8(0);
        CANVector(5) = bitand(uint8(Length), uint8(15));
        for i = 1:8
            CANVector(5+i) = uint8(Data(i));
        end
        RTSByte = uint8(RTS);
        WriteInstruction = uint8(0x02);
    else
        CANVector = zeros(1,13,'uint8');
        RTSByte = uint8(RTS);
        WriteInstruction = uint8(0x03);
    end

    count = count + uint16(1);
    if count >= uint16(period)
        count = uint16(0);
    end
else
    CANVector = zeros(1,13,'uint8');
    RTSByte = uint8(0x03);
    WriteInstruction = uint8(0x03);
    % don't increment count while MCP not ready
end

== matlab function ENV_scheduled/CAN Tx19/MATLAB Function ==
  settings: updateMethod=DISCRETE  sampleTime=.001
  data: WriteInstruction output; ID input uint32; CANVector output uint8; Length input uint8; Data input uint8; RTS input; RTSByte output; period input; offset input; MCPInitialized input
function [WriteInstruction, CANVector, RTSByte] = ConvertToVector(ID, Length, Data, RTS, period, offset, MCPInitialized)
%#codegen
persistent count;
if isempty(count)
    count = uint16(0);
end

if MCPInitialized
    if count == uint16(8)
        id_u16 = uint16(ID);
        CANVector = zeros(1,13,'uint8');
        CANVector(1) = uint8(bitshift(id_u16, -3));
        CANVector(2) = uint8(bitshift(bitand(id_u16, uint16(7)), 5));
        CANVector(3) = uint8(0);
        CANVector(4) = uint8(0);
        CANVector(5) = bitand(uint8(Length), uint8(15));
        for i = 1:8
            CANVector(5+i) = uint8(Data(i));
        end
        RTSByte = uint8(RTS);
        WriteInstruction = uint8(0x02);
    else
        CANVector = zeros(1,13,'uint8');
        RTSByte = uint8(RTS);
        WriteInstruction = uint8(0x03);
    end

    count = count + uint16(1);
    if count >= uint16(period)
        count = uint16(0);
    end
else
    CANVector = zeros(1,13,'uint8');
    RTSByte = uint8(0x03);
    WriteInstruction = uint8(0x03);
    % don't increment count while MCP not ready
end

== matlab function ENV_scheduled/CAN Rx/MATLAB Function ==
  data: RxBytes input uint8 size=14; Message output Bus: CAN_MESSAGE_def
function Message = DecodeCANMsg(RxBytes)
%#codegen

% rxBytes is uint8(1x14); byte 1 is the command echo (don't care)
SIDH = RxBytes(2);
SIDL = RxBytes(3);
EID8 = RxBytes(4);  %#ok — not used for standard frames
EID0 = RxBytes(5);  %#ok
DLC  = RxBytes(6);

% Assemble standard 11-bit ID
Message.ID       = uint32(bitor(uint32(bitshift(uint32(SIDH), 3)), ...
                            uint32(bitshift(uint32(SIDL), -5))));
Message.Extended = false;
Message.Remote   = false;
Message.Error    = false;
Message.Length   = double(bitand(DLC, uint8(15)));
Message.Data     = RxBytes(7:14);

== matlab function ENV_scheduled/CAN Tx/MATLAB Function ==
  settings: updateMethod=DISCRETE  sampleTime=.001
  data: WriteInstruction output; ID input uint32; CANVector output uint8; Length input uint8; Data input uint8; RTS input; RTSByte output; period input; offset input; MCPInitialized input
function [WriteInstruction, CANVector, RTSByte] = ConvertToVector(ID, Length, Data, RTS, period, offset, MCPInitialized)
%#codegen
persistent count;
if isempty(count)
    count = uint16(0);
end

if MCPInitialized
    if count == uint16(offset)
        id_u16 = uint16(ID);
        CANVector = zeros(1,13,'uint8');
        CANVector(1) = uint8(bitshift(id_u16, -3));
        CANVector(2) = uint8(bitshift(bitand(id_u16, uint16(7)), 5));
        CANVector(3) = uint8(0);
        CANVector(4) = uint8(0);
        CANVector(5) = bitand(uint8(Length), uint8(15));
        for i = 1:8
            CANVector(5+i) = uint8(Data(i));
        end
        RTSByte = uint8(RTS);
        WriteInstruction = uint8(0x02);
    else
        CANVector = zeros(1,13,'uint8');
        RTSByte = uint8(RTS);
        WriteInstruction = uint8(0x03);
    end

    count = count + uint16(1);
    if count >= uint16(period)
        count = uint16(0);
    end
else
    CANVector = zeros(1,13,'uint8');
    RTSByte = uint8(0x03);
    WriteInstruction = uint8(0x03);
    % don't increment count while MCP not ready
end

== matlab function ENV_scheduled/CAN Rx/MATLAB Function1 ==
  data: RxBytes input uint8 size=14; Message output Bus: CAN_MESSAGE_def
function Message = DecodeCANMsg(RxBytes)
%#codegen

% rxBytes is uint8(1x14); byte 1 is the command echo (don't care)
SIDH = RxBytes(2);
SIDL = RxBytes(3);
EID8 = RxBytes(4);  %#ok — not used for standard frames
EID0 = RxBytes(5);  %#ok
DLC  = RxBytes(6);

% Assemble standard 11-bit ID
Message.ID       = uint32(bitor(uint32(bitshift(uint32(SIDH), 3)), ...
                            uint32(bitshift(uint32(SIDL), -5))));
Message.Extended = false;
Message.Remote   = false;
Message.Error    = false;
Message.Length   = double(bitand(DLC, uint8(15)));
Message.Data     = RxBytes(7:14);

== matlab function ENV_scheduled/CAN Rx/MATLAB Function2 ==
  data: RxBytes input uint8 size=14; Message output Bus: CAN_MESSAGE_def
function Message = DecodeCANMsg(RxBytes)
%#codegen

% rxBytes is uint8(1x14); byte 1 is the command echo (don't care)
SIDH = RxBytes(2);
SIDL = RxBytes(3);
EID8 = RxBytes(4);  %#ok — not used for standard frames
EID0 = RxBytes(5);  %#ok
DLC  = RxBytes(6);

% Assemble standard 11-bit ID
Message.ID       = uint32(bitor(uint32(bitshift(uint32(SIDH), 3)), ...
                            uint32(bitshift(uint32(SIDL), -5))));
Message.Extended = false;
Message.Remote   = false;
Message.Error    = false;
Message.Length   = double(bitand(DLC, uint8(15)));
Message.Data     = RxBytes(7:14);

== matlab function ENV_scheduled/CAN Rx/MATLAB Function3 ==
  data: RxBytes input uint8 size=14; Message output Bus: CAN_MESSAGE_def
function Message = DecodeCANMsg(RxBytes)
%#codegen

% rxBytes is uint8(1x14); byte 1 is the command echo (don't care)
SIDH = RxBytes(2);
SIDL = RxBytes(3);
EID8 = RxBytes(4);  %#ok — not used for standard frames
EID0 = RxBytes(5);  %#ok
DLC  = RxBytes(6);

% Assemble standard 11-bit ID
Message.ID       = uint32(bitor(uint32(bitshift(uint32(SIDH), 3)), ...
                            uint32(bitshift(uint32(SIDL), -5))));
Message.Extended = false;
Message.Remote   = false;
Message.Error    = false;
Message.Length   = double(bitand(DLC, uint8(15)));
Message.Data     = RxBytes(7:14);

== matlab function ENV_scheduled/CAN Rx/MATLAB Function4 ==
  data: RxBytes input uint8 size=14; Message output Bus: CAN_MESSAGE_def
function Message = DecodeCANMsg(RxBytes)
%#codegen

% rxBytes is uint8(1x14); byte 1 is the command echo (don't care)
SIDH = RxBytes(2);
SIDL = RxBytes(3);
EID8 = RxBytes(4);  %#ok — not used for standard frames
EID0 = RxBytes(5);  %#ok
DLC  = RxBytes(6);

% Assemble standard 11-bit ID
Message.ID       = uint32(bitor(uint32(bitshift(uint32(SIDH), 3)), ...
                            uint32(bitshift(uint32(SIDL), -5))));
Message.Extended = false;
Message.Remote   = false;
Message.Error    = false;
Message.Length   = double(bitand(DLC, uint8(15)));
Message.Data     = RxBytes(7:14);

== matlab function ENV_scheduled/CAN Rx/MATLAB Function5 ==
  data: RxBytes input uint8 size=14; Message output Bus: CAN_MESSAGE_def
function Message = DecodeCANMsg(RxBytes)
%#codegen

% rxBytes is uint8(1x14); byte 1 is the command echo (don't care)
SIDH = RxBytes(2);
SIDL = RxBytes(3);
EID8 = RxBytes(4);  %#ok — not used for standard frames
EID0 = RxBytes(5);  %#ok
DLC  = RxBytes(6);

% Assemble standard 11-bit ID
Message.ID       = uint32(bitor(uint32(bitshift(uint32(SIDH), 3)), ...
                            uint32(bitshift(uint32(SIDL), -5))));
Message.Extended = false;
Message.Remote   = false;
Message.Error    = false;
Message.Length   = double(bitand(DLC, uint8(15)));
Message.Data     = RxBytes(7:14);

== matlab function ENV_scheduled/CAN Rx/MATLAB Function6 ==
  data: RxBytes input uint8 size=14; Message output Bus: CAN_MESSAGE_def
function Message = DecodeCANMsg(RxBytes)
%#codegen

% rxBytes is uint8(1x14); byte 1 is the command echo (don't care)
SIDH = RxBytes(2);
SIDL = RxBytes(3);
EID8 = RxBytes(4);  %#ok — not used for standard frames
EID0 = RxBytes(5);  %#ok
DLC  = RxBytes(6);

% Assemble standard 11-bit ID
Message.ID       = uint32(bitor(uint32(bitshift(uint32(SIDH), 3)), ...
                            uint32(bitshift(uint32(SIDL), -5))));
Message.Extended = false;
Message.Remote   = false;
Message.Error    = false;
Message.Length   = double(bitand(DLC, uint8(15)));
Message.Data     = RxBytes(7:14);
